simulink model "phase_discrimination"  (R2019b)
settings: Solver=VariableStepAuto  StartTime=0.0  StopTime=0.3  RelTol=1e-3
libraries: commsynccomp2 x1, cstblocks x1, dspsrcs4 x1
settings Model: Creator=Siddhartha  LastModifiedBy=Siddhartha

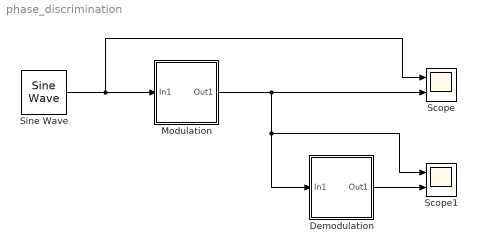
== system phase_discrimination ==
  "Demodulation " : Subsystem
  Modulation : Subsystem
  Scope : Scope  NumInputPorts=2
  Scope1 : Scope  NumInputPorts=2
  Sine Wave : dspsrcs4/Sine Wave  Amplitude=1  Frequency=10  Phase=0  SampleMode=Discrete  OutComplex=Real  CompMethod=Trigonometric fcn  TableSize=Speed  SampleTime=1/100000  SamplesPerFrame=1  ResetState=Restart at time zero  OutputFrames=off  dataType=double  wordLen=16  udDataType=sfix(16)  fracBitsMode=Best precision  numFracBits=15  OutDataTypeStr=double  LastOutDataTypeStr=double
  wires:
  Modulation/1(Out1) -> Scope/2, Scope1/1, "Demodulation "/1(In1)
  Sine Wave/1 -> Scope/1, Modulation/1(In1)
  "Demodulation "/1(Out1) -> Scope1/2

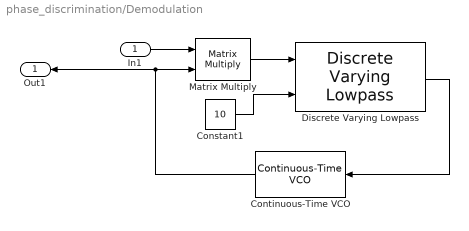
== system phase_discrimination/Demodulation  ==
  In1 : Inport
  Constant1 : Constant  Value=10
  Continuous-Time VCO : commsynccomp2/Continuous-Time VCO  Ac=1  Fc=10  Kc=1  Ph=0
      settings: SourceProductName=Communications Toolbox  SourceProductBaseCode=CM
  Discrete Varying Lowpass : cstblocks/Linear Parameter Varying/Discrete Varying Lowpass  N=5  w0=0  Ts=1
      settings: SourceProductName=Control System Toolbox  SourceProductBaseCode=CT
  Matrix Multiply : Product  Multiplication=Matrix(*)
  Out1 : Outport
  wires:
  Discrete Varying Lowpass/1 -> Continuous-Time VCO/1
  Constant1/1 -> Discrete Varying Lowpass/2
  In1/1 -> Matrix Multiply/1
  Matrix Multiply/1 -> Discrete Varying Lowpass/1
  Continuous-Time VCO/1 -> Out1/1, Matrix Multiply/2

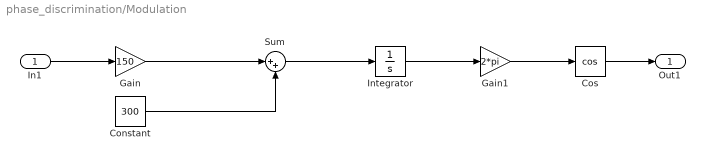
== system phase_discrimination/Modulation ==
  In1 : Inport
  Constant : Constant  Value=300
  Cos : Trigonometry  Operator=cos
  Gain : Gain  Gain=150
  Gain1 : Gain  Gain=2*pi
  Integrator : Integrator
  Sum : Sum  Inputs=|++
  Out1 : Outport
  wires:
  Integrator/1 -> Gain1/1
  Gain/1 -> Sum/1
  In1/1 -> Gain/1
  Constant/1 -> Sum/2
  Sum/1 -> Integrator/1
  Gain1/1 -> Cos/1
  Cos/1 -> Out1/1
